simulink model "test_libMdl_RailwayToolbox"  (R2018a)
settings: Solver=FixedStepDiscrete  StartTime=0  StopTime=t_end  RelTol=1e-3
PreLoadFcn:
  | init_test_libMdl_RailwayToolbox
InitFcn:
  | init_test_libMdl_RailwayToolbox
values from neighbouring files (symbols this model uses):
  a_train_0 = 0    [init_test_libMdl_RailwayToolbox.m]
  Q_kf = Gamma*sigma_v_kf.^2*Gamma'    [init_test_libMdl_RailwayToolbox.m]
  R_kf = diag(sigma_w_kf.^2)    [init_test_libMdl_RailwayToolbox.m]
  sigma_w_ref = [sigma_w_gps_ref; sigma_w_gps_ref; sigma_w_acc_ref; sigma_w_gyro_ref]    [init_test_libMdl_RailwayToolbox.m]
  v_train_0 = v_train_desired_kmh/3.6    (= 55.5555555556)    [init_test_libMdl_RailwayToolbox.m]
  v_train_desired_kmh = 200    [init_test_libMdl_RailwayToolbox.m]
  z_0_meas = [z_gps_0; z_acc_0; z_gyro_0]    [init_test_libMdl_RailwayToolbox.m]
libraries: libMdl_KalmanFilter x1, libMdl_TrainFrontDataGenerator x1, libMdl_Gnss x1, libMdl_Imu x1
settings Model: SimulationMode=accelerator  PauseTimes=224  Creator=hwinter  LastModifiedBy=hwinter
settings DataIOCC: SaveOutput=off  SignalLogging=off  DSMLogging=off  SaveTime=off
settings DebuggingCC: ReadBeforeWriteMsg=DisableAll  WriteAfterWriteMsg=DisableAll  WriteAfterReadMsg=DisableAll  MultiTaskDSMMsg=none
settings HardwareCC: ProdBitPerLong=64  ProdHWDeviceType=Intel->x86-64 (Linux 64)  TargetBitPerLong=64  TargetBitPerPointer=64  TargetBitPerSizeT=64  TargetBitPerPtrDiffT=64  TargetLongLongMode=on  TargetIntDivRoundTo=Zero  TargetEndianess=LittleEndian  TargetWordSize=64  TargetHWDeviceType=MATLAB Host  ProdEqTarget=off
settings SFSimCC: SFSimEcho=off
settings RTWCC: SystemTargetFile=rsim.tlc  TemplateMakefile=rsim_default_tmf  Description=Rapid Simulation Target
settings CodeAppCC: StateflowObjectComments=on
settings RSimTargetCC: TargetLangStandard=C99 (ISO)  GeneratePreprocessorConditionals=Use local settings

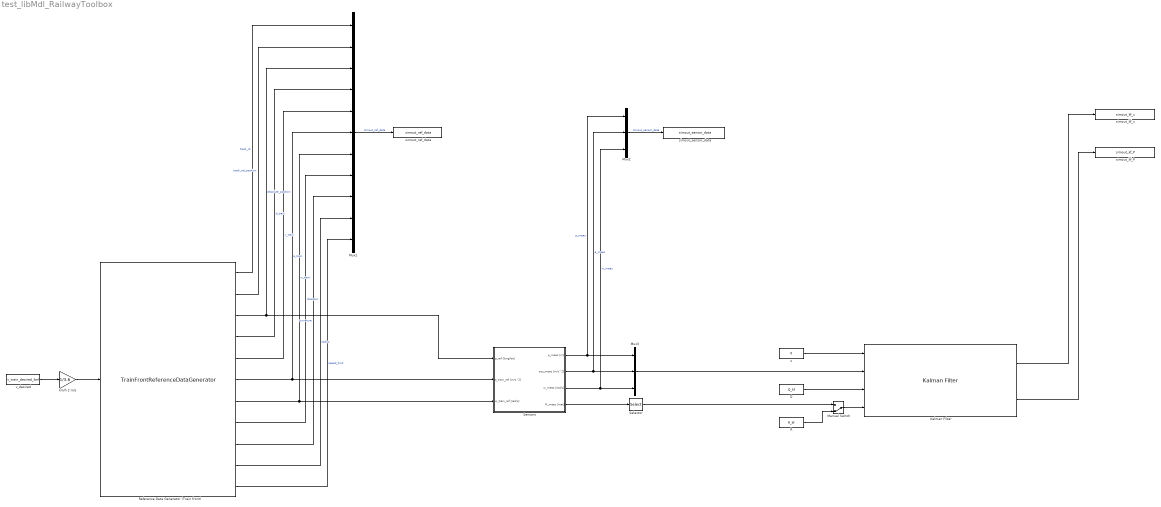
== system test_libMdl_RailwayToolbox ==
  Kalman Filter : libMdl_KalmanFilter/Kalman Filter  mv_sample_time=T_system  mv_x_0=x_0_kf  mv_P_0=P_0_kf  mv_state_transition_function=simFcn_test_libMdl_DataGenerator_StateTransitionFcn  mv_measurement_function=simFcn_test_libMdl_DataGenerator_MeasurementFcn
  Manual Switch : ManualSwitch  CurrentSetting=0
  Mux1 : Mux  Inputs=11
  Mux2 : Mux  Inputs=3
  Mux3 : Mux  Inputs=3
  Q : Constant  Value=Q_kf
  R : Constant  Value=R_kf
  Reference Data Generator (Train front) : libMdl_TrainFrontDataGenerator/TrainFrontReferenceDataGenerator  mv_T_ref_system=T_system  mv_motion_t_constant=1  mv_a_train_limits=max_train_acc  mv_track_id_0=track_id_0  mv_track_rel_position_0=track_rel_position_0  mv_x_0=[v_train_0, a_train_0]  mv_track_map=mat_track_map  mv_track_map_rot_angle=phi_track
  Selector : Selector  NumberOfDimensions=2  InputPortWidth=3  IndexOptions=Index vector (dialog),Index vector (dialog)  Indices=[1 2 3 8],[1 2 3 8]  OutputSizes=1,1
  Sensors : Subsystem
  km/h 2 m/s : Gain  Gain=1/3.6
  simout_kf_P : ToWorkspace  VariableName=simout_kf_P  SaveFormat=Timeseries  SampleTime=-1
  simout_kf_x : ToWorkspace  VariableName=simout_kf_x  SaveFormat=Timeseries  SampleTime=-1
  simout_ref_data : ToWorkspace  VariableName=simout_ref_data  SaveFormat=Timeseries  SampleTime=-1
  simout_sensor_data : ToWorkspace  VariableName=simout_sensor_data  SaveFormat=Timeseries  SampleTime=-1
  u : Constant  Value=0
  v_desired : Constant  Value=v_train_desired_kmh
  wires:
  Mux3/1 -> Kalman Filter/2
  v_desired/1 -> km/h 2 m/s/1
  Kalman Filter/1 -> simout_kf_x/1
  Kalman Filter/2 -> simout_kf_P/1
  Q/1 -> Kalman Filter/3
  u/1 -> Kalman Filter/1
  Manual Switch/1 -> Kalman Filter/4
  R/1 -> Manual Switch/2
  Selector/1 -> Manual Switch/1
  Reference Data Generator (Train front)/6 -> Mux1/6, Sensors/2(a_train_ref [m/s^2])  "a_train"
  Reference Data Generator (Train front)/7 -> Mux1/7, Sensors/3(w_train_ref [rad/s])  "w_train"
  Reference Data Generator (Train front)/3 -> Mux1/3, Sensors/1(p_ref [long/lat])  "absolute_position"
  km/h 2 m/s/1 -> Reference Data Generator (Train front)/1
  Sensors/1(p_meas [m]) -> Mux2/1, Mux3/1  "p_meas"
  Sensors/2(acc_meas [m/s^2]) -> Mux2/2, Mux3/2  "a_meas"
  Sensors/4(R_meas [mat]) -> Selector/1
  Reference Data Generator (Train front)/11 -> Mux1/11  "speed_limit"
  Reference Data Generator (Train front)/10 -> Mux1/10  "radius"
  Reference Data Generator (Train front)/9 -> Mux1/9  "curvature"
  Reference Data Generator (Train front)/8 -> Mux1/8  "direction"
  Reference Data Generator (Train front)/5 -> Mux1/5  "v_train"
  Reference Data Generator (Train front)/4 -> Mux1/4  "d_train"
  Reference Data Generator (Train front)/2 -> Mux1/2  "track_rel_position"
  Reference Data Generator (Train front)/1 -> Mux1/1  "track_id"
  Mux1/1 -> simout_ref_data/1  "simout_ref_data"
  Mux2/1 -> simout_sensor_data/1  "simout_sensor_data"
  Sensors/3(w_meas [rad/s]) -> Mux3/3, Mux2/3  "w_meas"

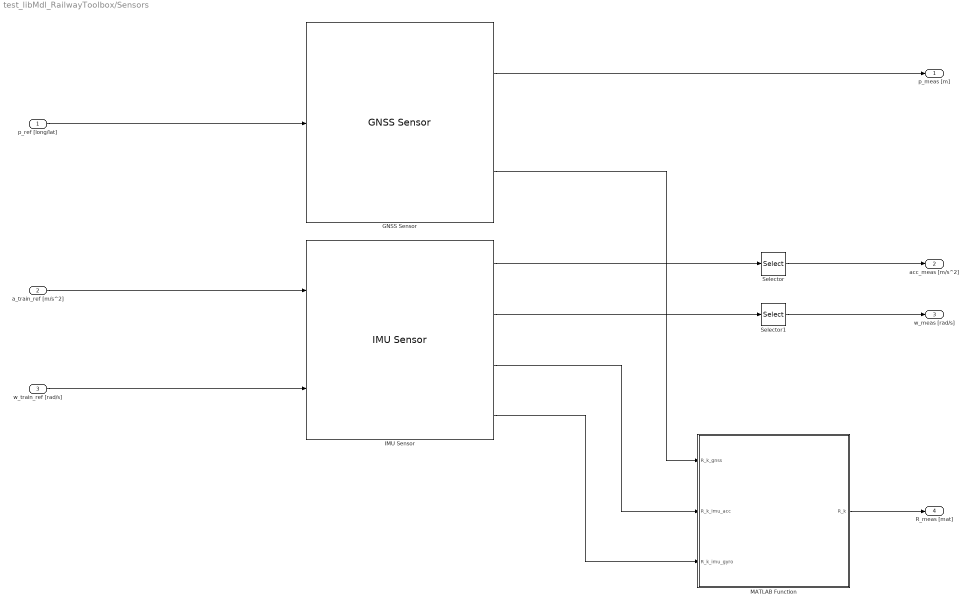
== system test_libMdl_RailwayToolbox/Sensors ==
  p_ref [long/lat] : Inport
  a_train_ref [m/s^2] : Inport  Port=2
  w_train_ref [rad/s] : Inport  Port=3
  GNSS Sensor : libMdl_Gnss/GNSS Sensor  mv_T_gnss=T_meas  mv_sigma_gnss=[sigma_w_ref(1), sigma_w_ref(2)]  mv_z_0_gnss=[z_0_meas(1), z_0_meas(2)]  mv_seed_gnss=gnss_rng_seed
  IMU Sensor : libMdl_Imu/IMU Sensor  mv_T_imu=T_meas  mv_sigma_imu_acc=[sigma_w_ref(3), sigma_w_ref(3), sigma_w_ref(3)]  mv_sigma_imu_gyro=[sigma_w_ref(4), sigma_w_ref(4), sigma_w_ref(4)]  mv_z_0_imu_acc=[z_0_meas(3), z_0_meas(3), z_0_meas(3)]  mv_z_0_imu_gyro=[z_0_meas(4), z_0_meas(4), z_0_meas(4)]  mv_seed_imu=imu_rng_seed
  MATLAB Function : MATLAB Function  TreatAsAtomicUnit=on
  Selector : Selector  InputPortWidth=3  IndexOptions=Index vector (dialog)  Indices=1  OutputSizes=1
  Selector1 : Selector  InputPortWidth=3  IndexOptions=Index vector (dialog)  Indices=3  OutputSizes=1
  p_meas [m] : Outport
  acc_meas [m/s^2] : Outport  Port=2
  w_meas [rad/s] : Outport  Port=3
  R_meas [mat] : Outport  Port=4
  wires:
  p_ref [long/lat]/1 -> GNSS Sensor/1
  GNSS Sensor/2 -> MATLAB Function/1(R_k_gnss)
  GNSS Sensor/1 -> p_meas [m]/1
  Selector1/1 -> w_meas [rad/s]/1
  Selector/1 -> acc_meas [m/s^2]/1
  IMU Sensor/1 -> Selector/1
  IMU Sensor/2 -> Selector1/1
  IMU Sensor/3 -> MATLAB Function/2(R_k_imu_acc)
  IMU Sensor/4 -> MATLAB Function/3(R_k_imu_gyro)
  w_train_ref [rad/s]/1 -> IMU Sensor/2
  MATLAB Function/1(R_k) -> R_meas [mat]/1
  a_train_ref [m/s^2]/1 -> IMU Sensor/1

== matlab function test_libMdl_RailwayToolbox/Sensors/MATLAB Function ==
  data: R_k_gnss input; R_k output; R_k_imu_acc input; R_k_imu_gyro input
function R_k = simFcn_createMeasurementCovarianceMatrix(R_k_gnss,R_k_imu_acc,R_k_imu_gyro)

R_k = blkdiag(R_k_gnss,R_k_imu_acc,R_k_imu_gyro);

end
